simulink model "cf_model"  (R2016a)
settings: Solver=VariableStepAuto  StartTime=0.0  StopTime=10  FixedStep=dt  RelTol=1e-3
values from neighbouring files (symbols this model uses):
  ic = [-3 0 0 0 0 0 0 0 0 0 0 0]    [cf_pid_compare.m]    (also in main.m = [0 0 0 0 0 0 0 0 0 0 0 0])
  r2d = 180/pi    (= 57.2957795131)    [main.m]
undefined symbols (not defined in the file or in its folder): default_ctl, est, geometric_ctl
undefined symbols (not defined in the file): cf2, pid_ctl
libraries: simulink x11, vrlib x8, aerolibtransform2 x8, aerolibutil x5, cstblocks x4, aerolibnav x2, dspmathops x2
(part 2 of 2)

== system cf_model/PID/PID Controller/Rate Control/PID1 ==
  Desired : Inport
  Measured : Inport  Port=2
  Add : Sum  Inputs=3
  Derivative : Derivative
  Integrator Limited : Integrator  LimitOutput=on  UpperSaturationLimit=intSat(3,2)  LowerSaturationLimit=-intSat(3,2)
  Kd : Gain  Gain=rates(2,3)  OutMin=[-200]  OutMax=[200]
  Ki : Gain  Gain=rates(2,2)  OutMin=[-200]  OutMax=[200]
  Kp : Gain  Gain=rates(2,1)  OutMin=[-200]  OutMax=[200]
  Subtract : Sum  Inputs=+-
  Output : Outport
  wires:
  Derivative/1 -> Kd/1
  Integrator Limited/1 -> Ki/1
  Subtract/1 -> Derivative/1, Integrator Limited/1, Kp/1
  Kd/1 -> Add/3
  Kp/1 -> Add/1
  Add/1 -> Output/1
  Ki/1 -> Add/2
  Desired/1 -> Subtract/1
  Measured/1 -> Subtract/2

== system cf_model/PID/PID Controller/Rate Control/PID2 ==
  Desired : Inport
  Measured : Inport  Port=2
  Add : Sum  Inputs=3
  Derivative : Derivative
  Integrator Limited : Integrator  LimitOutput=on  UpperSaturationLimit=intSat(3,3)  LowerSaturationLimit=-intSat(3,3)
  Kd : Gain  Gain=rates(3,3)  OutMin=[-200]  OutMax=[200]
  Ki : Gain  Gain=rates(3,2)  OutMin=[-200]  OutMax=[200]
  Kp : Gain  Gain=rates(3,1)  OutMin=[-200]  OutMax=[200]
  Subtract : Sum  Inputs=+-
  Output : Outport
  wires:
  Measured/1 -> Subtract/2
  Desired/1 -> Subtract/1
  Ki/1 -> Add/2
  Add/1 -> Output/1
  Kp/1 -> Add/1
  Kd/1 -> Add/3
  Subtract/1 -> Kp/1, Integrator Limited/1, Derivative/1
  Integrator Limited/1 -> Ki/1
  Derivative/1 -> Kd/1

== matlab function cf_model/PID/Vehicle/Vehicle Dynamics/MATLAB Function ==
  data: uvw input; xyz_dot output; angles input
function xyz_dot  = Position(uvw,angles)
xyz_dot = zeros(3,1);
phi = angles(1); %*pi/180;
theta = angles(2); %*pi/180;
psi = angles(3); %*pi/180;
Tb_o = [cos(theta)*cos(psi)                                cos(theta)*sin(psi)                             -sin(theta)  ;   %BBF > Inertial rotation matrix
        sin(phi)*sin(theta)*cos(psi)-cos(phi)*sin(psi)    sin(phi)*sin(theta)*sin(psi)+cos(phi)*cos(psi)  sin(phi)*cos(theta) ;
        cos(phi)*sin(theta)*cos(psi)+sin(phi)*sin(psi)    cos(phi)*sin(theta)*sin(psi)-sin(phi)*cos(psi)   cos(phi)*cos(theta)];

xyz_dot = (Tb_o')*uvw;
end

== matlab function cf_model/PID/PID Controller/MATLAB Function1 ==
  data: position input; position_error output; desired_position input
function position_error  = world_error(position,desired_position)
%#Position Error in world Frame
position_error = [0;0;0];


position_error = [desired_position(1)-position(1);...
                  desired_position(2)-position(2);...
                  desired_position(3)-position(3)];

end

== matlab function cf_model/PID/Vehicle/Vehicle Dynamics/MATLAB Function1 ==
  data: pqr input; angles_dot output; angles input
function angles_dot  = Angle(pqr,angles)
angles_dot = zeros(3,1);
phi = angles(1); %*pi/180;
theta = angles(2); %*pi/180;

H = [1    sin(phi)*tan(theta)     cos(phi)*tan(theta)
     0       cos(phi)                 -sin(phi)   
     0       sin(phi)/cos(theta)    cos(phi)/cos(theta)];
angles_dot = H*pqr;
end

== matlab function cf_model/circle /Calc_Omg_des  ==
  data: a_des input; omg_des output; j_des input; s_des input; yaw_des input; dyaw_des input; ddyaw_des input; omg_des_dot output
function [omg_des, omg_des_dot]= fcn(a_des, j_des, s_des, yaw_des, dyaw_des, ddyaw_des)
thrust = a_des+[0 0 9.81]';
u1_m = norm(thrust);
z_b = thrust/u1_m;
x_w = [cos(yaw_des) sin(yaw_des) 0];
y_b = cross(z_b, x_w);
y_b = y_b/norm(y_b);
x_b = cross(y_b, z_b);

u1_dot_m = dot(z_b, j_des);
h_w = (j_des - u1_dot_m*z_b)/u1_m;

p = -dot(h_w, y_b);
q = dot(h_w, x_b);
r = dyaw_des*z_b(3);
omg_des = [p q r]';

u1_ddot_m = dot(z_b, s_des) - dot(z_b, cross(omg_des, cross(omg_des, u1_m*z_b)));
h_a = (s_des - u1_ddot_m*z_b - 2*cross(omg_des, u1_dot_m*z_b) - cross(omg_des, cross(omg_des, u1_m*z_b)))/u1_m;

p_dot = -dot(h_a, y_b);
q_dot = dot(h_a, x_b);
r_dot = ddyaw_des*z_b(3);
omg_des_dot = [p_dot, q_dot, r_dot]';

== matlab function cf_model/PID/Vehicle/Vehicle Dynamics/MATLAB Function2 ==
  data: uvw input; uvw_dot output; pqr input; angles input; F input; model parameter
function uvw_dot  = Forces(uvw,pqr,angles,F,model)
uvw_dot = zeros(3,1);
drag = -uvw .* model.c_drag .* model.AirDensity .* model.a;

Force = [0;0;F]+drag;
g_o = [0;0;-9.81];

phi = angles(1); %*pi/180;
theta = angles(2); %*pi/180;
psi = angles(3); %*pi/180;
Tb_o = [cos(theta)*cos(psi)                                cos(theta)*sin(psi)                             -sin(theta)  ;   %BBF > Inertial rotation matrix
        sin(phi)*sin(theta)*cos(psi)-cos(phi)*sin(psi)    sin(phi)*sin(theta)*sin(psi)+cos(phi)*cos(psi)  sin(phi)*cos(theta) ;
        cos(phi)*sin(theta)*cos(psi)+sin(phi)*sin(psi)    cos(phi)*sin(theta)*sin(psi)-sin(phi)*cos(psi)   cos(phi)*cos(theta)];

uvw_dot = Force + Tb_o*g_o - cross(pqr,uvw);
 
end

== matlab function cf_model/PID/Vehicle/Vehicle Dynamics/MATLAB Function3 ==
  data: pqr_dot output; pqr input; M input
function pqr_dot  = Moments(pqr,M)
pqr_dot = zeros(3,1);
Ixx =  1.395e-05;  %2.3951e-5; %1.39e-05; %2.51943e-5; % % %
Iyy = 1.436e-05; %2.3951e-5; %1.436e-05; % 2.54379e-5; % %         %
Izz =  2.173e-05;  %3.2347e-5; %2.173e-05 ; %4.51407e-5; % %         %;%0.160;
J = diag([Ixx Iyy Izz]);    %   I  Flyer rotational inertia matrix     3x3
pqr_dot = inv(J)*(M-cross(pqr,J*pqr));
end

== matlab function cf_model/PID/Estimator/Mahoney/calc v3 ==
  data: q input; v output
function v = fcn(q)
%#codegen
v = zeros(3,1);
v = [2*(q(2)*q(4) - q(1)*q(3))
         2*(q(1)*q(2) + q(3)*q(4))
         q(1)^2 - q(2)^2 - q(3)^2 + q(4)^2];
end

== matlab function cf_model/PID/Estimator/Mahoney/calc v ==
  data: q input; v output
function v = fcn(q)
%#codegen
v = zeros(3,1);
v = [2*(q(2)*q(4) - q(1)*q(3))
         2*(q(1)*q(2) + q(3)*q(4))
         q(1)^2 - q(2)^2 - q(3)^2 + q(4)^2];
end

== matlab function cf_model/PID/Estimator/Mahoney/quatprod ==
  data: a input; ab output; b input
function ab = quaternProd(a, b)
%QUATERNPROD Calculates the quaternion product
%
%   ab = quaternProd(a, b)
%
%   Calculates the quaternion product of quaternion a and b.
%
%   For more information see:
%   http://www.x-io.co.uk/node/8#quaternions
%
%	Date          Author          Notes
%	27/09/2011    SOH Madgwick    Initial release
    ab = zeros(1,4);
    ab(:,1) = a(:,1).*b(:,1)-a(:,2).*b(:,2)-a(:,3).*b(:,3)-a(:,4).*b(:,4);
    ab(:,2) = a(:,1).*b(:,2)+a(:,2).*b(:,1)+a(:,3).*b(:,4)-a(:,4).*b(:,3);
    ab(:,3) = a(:,1).*b(:,3)-a(:,2).*b(:,4)+a(:,3).*b(:,1)+a(:,4).*b(:,2);
    ab(:,4) = a(:,1).*b(:,4)+a(:,2).*b(:,3)-a(:,3).*b(:,2)+a(:,4).*b(:,1);
end

== matlab function cf_model/Estimator3/Mahony/calc v ==
  data: q input; v output
function v = fcn(q)
%#codegen
v = zeros(3,1);
v = [2*(q(2)*q(4) - q(1)*q(3))
         2*(q(1)*q(2) + q(3)*q(4))
         q(1)^2 - q(2)^2 - q(3)^2 + q(4)^2];
end

== matlab function cf_model/Estimator3/Mahony/calc v3 ==
  data: q input; v output
function v = fcn(q)
%#codegen
v = zeros(3,1);
v = [2*(q(2)*q(4) - q(1)*q(3))
         2*(q(1)*q(2) + q(3)*q(4))
         q(1)^2 - q(2)^2 - q(3)^2 + q(4)^2];
end

== matlab function cf_model/Estimator3/Mahony/quatprod ==
  data: a input; ab output; b input
function ab = quaternProd(a, b)
%QUATERNPROD Calculates the quaternion product
%
%   ab = quaternProd(a, b)
%
%   Calculates the quaternion product of quaternion a and b.
%
%   For more information see:
%   http://www.x-io.co.uk/node/8#quaternions
%
%	Date          Author          Notes
%	27/09/2011    SOH Madgwick    Initial release
    ab = zeros(1,4);
    ab(:,1) = a(:,1).*b(:,1)-a(:,2).*b(:,2)-a(:,3).*b(:,3)-a(:,4).*b(:,4);
    ab(:,2) = a(:,1).*b(:,2)+a(:,2).*b(:,1)+a(:,3).*b(:,4)-a(:,4).*b(:,3);
    ab(:,3) = a(:,1).*b(:,3)-a(:,2).*b(:,4)+a(:,3).*b(:,1)+a(:,4).*b(:,2);
    ab(:,4) = a(:,1).*b(:,4)+a(:,2).*b(:,3)-a(:,3).*b(:,2)+a(:,4).*b(:,1);
end

== matlab function cf_model/Vehicle3/Vehicle Dynamics/MATLAB Function ==
  data: uvw input; xyz_dot output; angles input
function xyz_dot  = Position(uvw,angles)
xyz_dot = zeros(3,1);
phi = angles(1); %*pi/180;
theta = angles(2); %*pi/180;
psi = angles(3); %*pi/180;
Tb_o = [cos(theta)*cos(psi)                                cos(theta)*sin(psi)                             -sin(theta)  ;   %BBF > Inertial rotation matrix
        sin(phi)*sin(theta)*cos(psi)-cos(phi)*sin(psi)    sin(phi)*sin(theta)*sin(psi)+cos(phi)*cos(psi)  sin(phi)*cos(theta) ;
        cos(phi)*sin(theta)*cos(psi)+sin(phi)*sin(psi)    cos(phi)*sin(theta)*sin(psi)-sin(phi)*cos(psi)   cos(phi)*cos(theta)];

xyz_dot = (Tb_o')*uvw;
end

== matlab function cf_model/Vehicle3/Vehicle Dynamics/MATLAB Function1 ==
  data: pqr input; angles_dot output; angles input
function angles_dot  = Angle(pqr,angles)
angles_dot = zeros(3,1);
phi = angles(1); %*pi/180;
theta = angles(2); %*pi/180;

H = [1    sin(phi)*tan(theta)     cos(phi)*tan(theta)
     0       cos(phi)                 -sin(phi)   
     0       sin(phi)/cos(theta)    cos(phi)/cos(theta)];
angles_dot = H*pqr;
end

== matlab function cf_model/Vehicle3/Vehicle Dynamics/MATLAB Function2 ==
  data: uvw input; uvw_dot output; pqr input; angles input; F input
function uvw_dot  = Forces(uvw,pqr,angles,F)
uvw_dot = zeros(3,1);
Force = [0;0;F];
g_o = [0;0;-9.81];
phi = angles(1); %*pi/180;
theta = angles(2); %*pi/180;
psi = angles(3); %*pi/180;
Tb_o = [cos(theta)*cos(psi)                                cos(theta)*sin(psi)                             -sin(theta)  ;   %BBF > Inertial rotation matrix
        sin(phi)*sin(theta)*cos(psi)-cos(phi)*sin(psi)    sin(phi)*sin(theta)*sin(psi)+cos(phi)*cos(psi)  sin(phi)*cos(theta) ;
        cos(phi)*sin(theta)*cos(psi)+sin(phi)*sin(psi)    cos(phi)*sin(theta)*sin(psi)-sin(phi)*cos(psi)   cos(phi)*cos(theta)];

uvw_dot = Force + Tb_o*g_o - cross(pqr,uvw);

end

== matlab function cf_model/Vehicle3/Vehicle Dynamics/MATLAB Function3 ==
  data: pqr_dot output; pqr input; M input
function pqr_dot  = Moments(pqr,M)
pqr_dot = zeros(3,1);
Ixx =  1.395e-05;  %2.3951e-5; %1.39e-05; %2.51943e-5; % % %
Iyy = 1.436e-05; %2.3951e-5; %1.436e-05; % 2.54379e-5; % %         %
Izz =  2.173e-05;  %3.2347e-5; %2.173e-05 ; %4.51407e-5; % %         %;%0.160;
J = diag([Ixx Iyy Izz]);    %   I  Flyer rotational inertia matrix     3x3
pqr_dot = inv(J)*(M-cross(pqr,J*pqr));
end
